simulink model "question1"  (R2019a)
settings: Solver=VariableStepAuto  StartTime=0.0  StopTime=3  RelTol=1e-3
libraries: fl_lib x69, nesl_utility x22
settings Model: Creator=11lot  LastModifiedBy=11lot

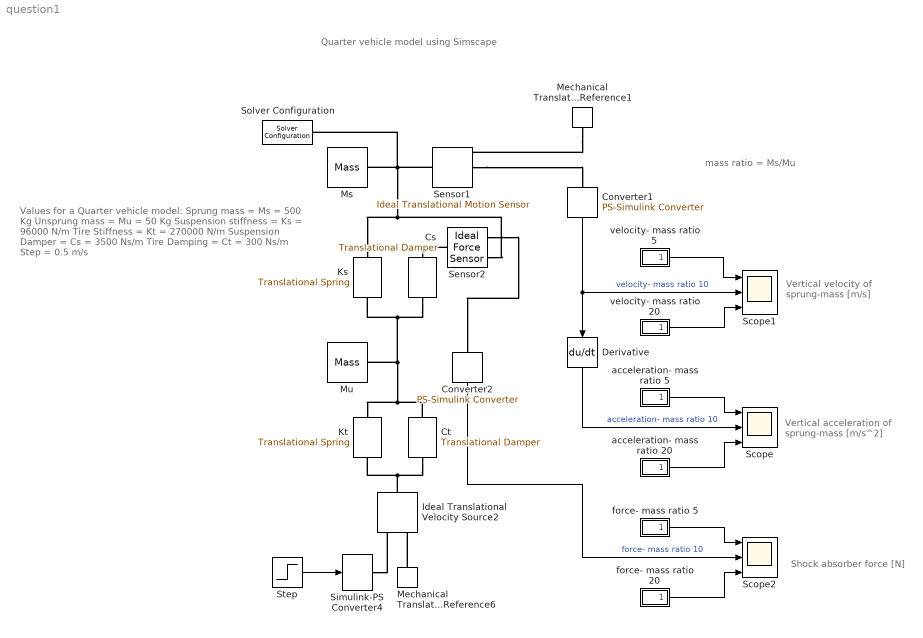
== system question1 ==
  note: mass ratio = Ms/Mu
  note: Values for a Quarter vehicle model:
      |
      | Sprung mass = Ms = 500 Kg
      | Unsprung mass = Mu = 50 Kg
      | Suspension stiffness = Ks = 96000 N/m
      | Tire Stiffness = Kt = 270000 N/m
      | Suspension Damper = Cs = 3500 Ns/m
      | Tire Damping = Ct = 300 Ns/m
      | Step = 0.5 m/s
  note: Quarter vehicle model using Simscape
  note: Vertical velocity of sprung-mass [m/s]
  note: Vertical acceleration of sprung-mass [m/s^2]
  note: Shock absorber force [N]
  " Ks" : fl_lib/Mechanical/Translational Elements/Translational Spring  spr_rate=96000 N/m  v_specify=off  v_priority=High  v=0 m/s  v_nominal_specify=off  v_nominal_unit=m/s  v_nominal_value=1  f_specify=off  f_priority=None  f=0 N  f_nominal_specify=off  f_nominal_unit=N  f_nominal_value=1  x_specify=on  x_priority=High  x=0 m  x_nominal_specify=off  x_nominal_unit=m  x_nominal_value=1
  " Kt" : fl_lib/Mechanical/Translational Elements/Translational Spring  spr_rate=270000 N/m  v_specify=off  v_priority=High  v=0 m/s  v_nominal_specify=off  v_nominal_unit=m/s  v_nominal_value=1  f_specify=off  f_priority=None  f=0 N  f_nominal_specify=off  f_nominal_unit=N  f_nominal_value=1  x_specify=on  x_priority=High  x=0 m  x_nominal_specify=off  x_nominal_unit=m  x_nominal_value=1
  " acceleration- mass ratio 20" : Subsystem
  " acceleration- mass ratio 5" : Subsystem
  Converter1 : nesl_utility/PS-Simulink Converter  PhysicalDomain=network_engine_domain  SubClassName=ps_output  LeftPortType=input  RightPortType=output  PseudoPeriodic=off  Frequencies=[]  Unit=m/s  AffineConversion=off
  Converter2 : nesl_utility/PS-Simulink Converter  PhysicalDomain=network_engine_domain  SubClassName=ps_output  LeftPortType=input  RightPortType=output  PseudoPeriodic=off  Frequencies=[]  Unit=N  AffineConversion=off
  Cs : fl_lib/Mechanical/Translational Elements/Translational Damper  D=3500 N/(m/s)  v_specify=off  v_priority=High  v=0 m/s  v_nominal_specify=off  v_nominal_unit=m/s  v_nominal_value=1  f_specify=off  f_priority=None  f=0 N  f_nominal_specify=off  f_nominal_unit=N  f_nominal_value=1
  Ct : fl_lib/Mechanical/Translational Elements/Translational Damper  D=300 N/(m/s)  v_specify=off  v_priority=High  v=0 m/s  v_nominal_specify=off  v_nominal_unit=m/s  v_nominal_value=1  f_specify=off  f_priority=None  f=0 N  f_nominal_specify=off  f_nominal_unit=N  f_nominal_value=1
  Derivative : Derivative
  Ideal Translational Velocity Source2 : fl_lib/Mechanical/Mechanical Sources/Ideal Translational Velocity Source
  Mechanical Translational Reference1 : fl_lib/Mechanical/Translational Elements/Mechanical Translational Reference
  Mechanical Translational Reference6 : fl_lib/Mechanical/Translational Elements/Mechanical Translational Reference
  Ms : fl_lib/Mechanical/Translational Elements/Mass  mass=500 kg  v_specify=on  v_priority=High  v=0 m/s  v_nominal_specify=off  v_nominal_unit=m/s  v_nominal_value=1  f_specify=off  f_priority=High  f=0 N  f_nominal_specify=off  f_nominal_unit=N  f_nominal_value=1
  Mu : fl_lib/Mechanical/Translational Elements/Mass  mass=50 kg  v_specify=on  v_priority=High  v=0 m/s  v_nominal_specify=off  v_nominal_unit=m/s  v_nominal_value=1  f_specify=off  f_priority=High  f=0 N  f_nominal_specify=off  f_nominal_unit=N  f_nominal_value=1
  Scope : Scope  NumInputPorts=3
  Scope1 : Scope  NumInputPorts=3
  Scope2 : Scope  NumInputPorts=3
  Sensor1 : fl_lib/Mechanical/Mechanical Sensors/Ideal Translational Motion Sensor  offset=0 m
  Sensor2 : fl_lib/Mechanical/Mechanical Sensors/Ideal Force Sensor
  Simulink-PS Converter4 : nesl_utility/Simulink-PS Converter  PhysicalDomain=network_engine_domain  SubClassName=ps_input  LeftPortType=input  RightPortType=output  PseudoPeriodic=off  Frequencies=[]  NoiseDistribution=none  NoiseParameters=[]  Unit=m/s  AffineConversion=off  FilteringAndDerivatives=zero  SimscapeFilterOrder=1  InputFilterTimeConstant=.001  UdotUserProvided=1
  Solver Configuration : nesl_utility/Solver Configuration  PhysicalDomain=network_engine_domain  SubClassName=solver  LeftPortType=input  RightPortType=generic  Tones=[]  Harmonics=[]  SimulateNoise=off  Profile=off  UseLocalSampling=off  EnableSwitchedLinearOptims=on  FrequencyDomain=off  UseCCode=off  RelTol=0.001  AbsTol=1e-06  MinStep=1e-09  ToWorkspace=off  RevertToSquareIcSolve=off  NumHomotopyIterations=100  PhasorMode=off  PhasorModeNumHarmonics=1  DoDC=off  ResidualTolerance=1e-9  UseLocalSolver=off  LocalSolverChoice=NE_BACKWARD_EULER_ADVANCER  LocalSolverSampleTime=.001  DoFixedCost=off  MaxNonlinIter=12  MaxModeIter=2  LinearAlgebra=Sparse  EquationFormulation=NE_TIME_EF  DelaysMemoryBudget=1024  AutomaticFiltering=on  FilteringTimeConstant=0.001  PartitionStorageMethod=AS_NEEDED  PartitionMemoryBudget=1024  PartitionMethod=FAST
  Step : Step  Time=0  After=0.5  SampleTime=0
  force- mass ratio 20 : Subsystem
  force- mass ratio 5 : Subsystem
  velocity- mass ratio 20 : Subsystem
  velocity- mass ratio 5 : Subsystem
  wires:
  Step/1 -> Simulink-PS Converter4/1
  Converter1/1 -> Derivative/1, Scope1/2  "velocity- mass ratio 10"
  Derivative/1 -> Scope/2  "acceleration- mass ratio 10"
  velocity- mass ratio 5/1(Out1) -> Scope1/1
  velocity- mass ratio 20/1(Out2) -> Scope1/3
  " acceleration- mass ratio 5"/1(Out1) -> Scope/1
  " acceleration- mass ratio 20"/1(Out1) -> Scope/3
  Converter2/1 -> Scope2/2  "force- mass ratio 10"
  force- mass ratio 5/1(Out1) -> Scope2/1
  force- mass ratio 20/1(Out1) -> Scope2/3
  connections:
  " Ks"/RConn1 -- Ct/LConn1 -- " Kt"/LConn1 -- Mu/LConn1 -- Cs/RConn1
  Ideal Translational Velocity Source2/LConn1 -- Ct/RConn1 -- " Kt"/RConn1
  Sensor1/LConn1 -- Solver Configuration/RConn1 -- Ms/LConn1 -- Sensor2/RConn1 -- " Ks"/LConn1
  Mechanical Translational Reference6/LConn1 -- Ideal Translational Velocity Source2/RConn2
  Simulink-PS Converter4/RConn1 -- Ideal Translational Velocity Source2/RConn1
  Mechanical Translational Reference1/LConn1 -- Sensor1/RConn1
  Sensor1/RConn2 -- Converter1/LConn1
  Sensor2/RConn2 -- Converter2/LConn1
  Sensor2/LConn1 -- Cs/LConn1

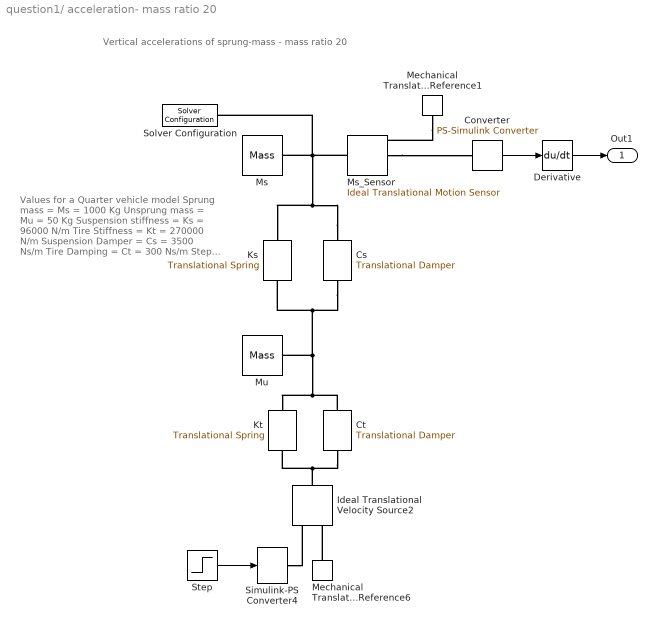
== system question1/ acceleration- mass ratio 20 ==
  note: Vertical accelerations of sprung-mass - mass ratio 20
  note: Values for a Quarter vehicle model
      |
      | Sprung mass = Ms = 1000 Kg
      | Unsprung mass = Mu = 50 Kg
      | Suspension stiffness = Ks = 96000 N/m
      | Tire Stiffness = Kt = 270000 N/m
      | Suspension Damper = Cs = 3500 Ns/m
      | Tire Damping = Ct = 300 Ns/m
      | Step = 0.5 m/s
  " Ms_Sensor" : fl_lib/Mechanical/Mechanical Sensors/Ideal Translational Motion Sensor  offset=0 m
  " Ks" : fl_lib/Mechanical/Translational Elements/Translational Spring  spr_rate=96000 N/m  v_specify=off  v_priority=None  v=0 m/s  v_nominal_specify=off  v_nominal_unit=m/s  v_nominal_value=1  f_specify=off  f_priority=None  f=0 N  f_nominal_specify=off  f_nominal_unit=N  f_nominal_value=1  x_specify=on  x_priority=High  x=0 m  x_nominal_specify=off  x_nominal_unit=m  x_nominal_value=1
  " Kt" : fl_lib/Mechanical/Translational Elements/Translational Spring  spr_rate=270000 N/m  v_specify=off  v_priority=None  v=0 m/s  v_nominal_specify=off  v_nominal_unit=m/s  v_nominal_value=1  f_specify=off  f_priority=None  f=0 N  f_nominal_specify=off  f_nominal_unit=N  f_nominal_value=1  x_specify=on  x_priority=High  x=0 m  x_nominal_specify=off  x_nominal_unit=m  x_nominal_value=1
  Converter : nesl_utility/PS-Simulink Converter  PhysicalDomain=network_engine_domain  SubClassName=ps_output  LeftPortType=input  RightPortType=output  PseudoPeriodic=off  Frequencies=[]  Unit=m/s  AffineConversion=off
  Cs : fl_lib/Mechanical/Translational Elements/Translational Damper  D=3500 N/(m/s)  v_specify=off  v_priority=None  v=0 m/s  v_nominal_specify=off  v_nominal_unit=m/s  v_nominal_value=1  f_specify=off  f_priority=None  f=0 N  f_nominal_specify=off  f_nominal_unit=N  f_nominal_value=1
  Ct : fl_lib/Mechanical/Translational Elements/Translational Damper  D=300 N/(m/s)  v_specify=off  v_priority=None  v=0 m/s  v_nominal_specify=off  v_nominal_unit=m/s  v_nominal_value=1  f_specify=off  f_priority=None  f=0 N  f_nominal_specify=off  f_nominal_unit=N  f_nominal_value=1
  Derivative : Derivative
  Ideal Translational Velocity Source2 : fl_lib/Mechanical/Mechanical Sources/Ideal Translational Velocity Source
  Mechanical Translational Reference1 : fl_lib/Mechanical/Translational Elements/Mechanical Translational Reference
  Mechanical Translational Reference6 : fl_lib/Mechanical/Translational Elements/Mechanical Translational Reference
  Ms : fl_lib/Mechanical/Translational Elements/Mass  mass=1000 kg  v_specify=on  v_priority=High  v=0 m/s  v_nominal_specify=off  v_nominal_unit=m/s  v_nominal_value=1  f_specify=off  f_priority=None  f=0 N  f_nominal_specify=off  f_nominal_unit=N  f_nominal_value=1
  Mu : fl_lib/Mechanical/Translational Elements/Mass  mass=50 kg  v_specify=on  v_priority=High  v=0 m/s  v_nominal_specify=off  v_nominal_unit=m/s  v_nominal_value=1  f_specify=off  f_priority=None  f=0 N  f_nominal_specify=off  f_nominal_unit=N  f_nominal_value=1
  Simulink-PS Converter4 : nesl_utility/Simulink-PS Converter  PhysicalDomain=network_engine_domain  SubClassName=ps_input  LeftPortType=input  RightPortType=output  PseudoPeriodic=off  Frequencies=[]  NoiseDistribution=none  NoiseParameters=[]  Unit=m/s  AffineConversion=off  FilteringAndDerivatives=zero  SimscapeFilterOrder=1  InputFilterTimeConstant=.001  UdotUserProvided=1
  Solver Configuration : nesl_utility/Solver Configuration  PhysicalDomain=network_engine_domain  SubClassName=solver  LeftPortType=input  RightPortType=generic  Tones=[]  Harmonics=[]  SimulateNoise=off  Profile=off  UseLocalSampling=off  EnableSwitchedLinearOptims=on  FrequencyDomain=off  UseCCode=off  RelTol=0.001  AbsTol=1e-06  MinStep=1e-09  ToWorkspace=off  RevertToSquareIcSolve=off  NumHomotopyIterations=100  PhasorMode=off  PhasorModeNumHarmonics=1  DoDC=off  ResidualTolerance=1e-9  UseLocalSolver=off  LocalSolverChoice=NE_BACKWARD_EULER_ADVANCER  LocalSolverSampleTime=.001  DoFixedCost=off  MaxNonlinIter=12  MaxModeIter=2  LinearAlgebra=Sparse  EquationFormulation=NE_TIME_EF  DelaysMemoryBudget=1024  AutomaticFiltering=on  FilteringTimeConstant=0.001  PartitionStorageMethod=AS_NEEDED  PartitionMemoryBudget=1024  PartitionMethod=FAST
  Step : Step  Time=0  After=0.5  SampleTime=0
  Out1 : Outport
  wires:
  Step/1 -> Simulink-PS Converter4/1
  Converter/1 -> Derivative/1
  Derivative/1 -> Out1/1
  connections:
  Ct/LConn1 -- " Kt"/LConn1 -- Mu/LConn1 -- Cs/RConn1 -- " Ks"/RConn1
  Cs/LConn1 -- " Ms_Sensor"/LConn1 -- Solver Configuration/RConn1 -- Ms/LConn1 -- " Ks"/LConn1
  " Kt"/RConn1 -- Ct/RConn1 -- Ideal Translational Velocity Source2/LConn1
  " Ms_Sensor"/RConn2 -- Converter/LConn1
  Mechanical Translational Reference1/LConn1 -- " Ms_Sensor"/RConn1
  Mechanical Translational Reference6/LConn1 -- Ideal Translational Velocity Source2/RConn2
  Simulink-PS Converter4/RConn1 -- Ideal Translational Velocity Source2/RConn1

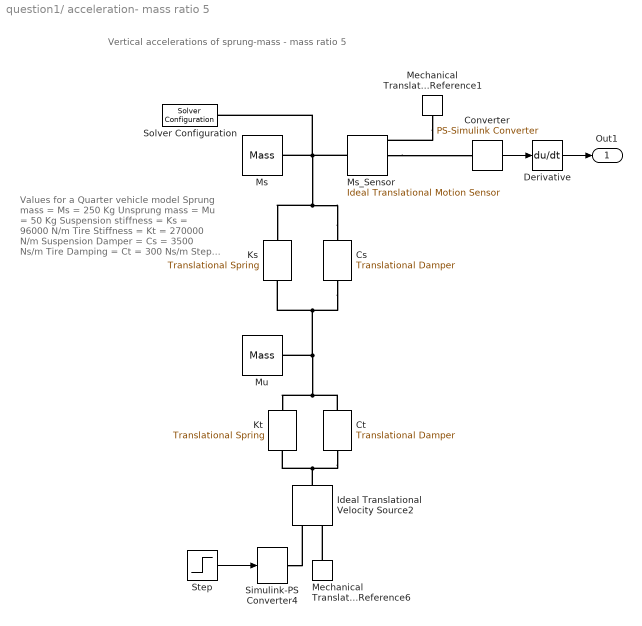
== system question1/ acceleration- mass ratio 5 ==
  note: Vertical accelerations of sprung-mass - mass ratio 5
  note: Values for a Quarter vehicle model
      |
      | Sprung mass = Ms = 250 Kg
      | Unsprung mass = Mu = 50 Kg
      | Suspension stiffness = Ks = 96000 N/m
      | Tire Stiffness = Kt = 270000 N/m
      | Suspension Damper = Cs = 3500 Ns/m
      | Tire Damping = Ct = 300 Ns/m
      | Step = 0.5 m/s
  " Ms_Sensor" : fl_lib/Mechanical/Mechanical Sensors/Ideal Translational Motion Sensor  offset=0 m
  " Ks" : fl_lib/Mechanical/Translational Elements/Translational Spring  spr_rate=96000 N/m  v_specify=off  v_priority=None  v=0 m/s  v_nominal_specify=off  v_nominal_unit=m/s  v_nominal_value=1  f_specify=off  f_priority=None  f=0 N  f_nominal_specify=off  f_nominal_unit=N  f_nominal_value=1  x_specify=on  x_priority=High  x=0 m  x_nominal_specify=off  x_nominal_unit=m  x_nominal_value=1
  " Kt" : fl_lib/Mechanical/Translational Elements/Translational Spring  spr_rate=270000 N/m  v_specify=off  v_priority=None  v=0 m/s  v_nominal_specify=off  v_nominal_unit=m/s  v_nominal_value=1  f_specify=off  f_priority=None  f=0 N  f_nominal_specify=off  f_nominal_unit=N  f_nominal_value=1  x_specify=on  x_priority=High  x=0 m  x_nominal_specify=off  x_nominal_unit=m  x_nominal_value=1
  Converter : nesl_utility/PS-Simulink Converter  PhysicalDomain=network_engine_domain  SubClassName=ps_output  LeftPortType=input  RightPortType=output  PseudoPeriodic=off  Frequencies=[]  Unit=m/s  AffineConversion=off
  Cs : fl_lib/Mechanical/Translational Elements/Translational Damper  D=3500 N/(m/s)  v_specify=off  v_priority=None  v=0 m/s  v_nominal_specify=off  v_nominal_unit=m/s  v_nominal_value=1  f_specify=off  f_priority=None  f=0 N  f_nominal_specify=off  f_nominal_unit=N  f_nominal_value=1
  Ct : fl_lib/Mechanical/Translational Elements/Translational Damper  D=300 N/(m/s)  v_specify=off  v_priority=None  v=0 m/s  v_nominal_specify=off  v_nominal_unit=m/s  v_nominal_value=1  f_specify=off  f_priority=None  f=0 N  f_nominal_specify=off  f_nominal_unit=N  f_nominal_value=1
  Derivative : Derivative
  Ideal Translational Velocity Source2 : fl_lib/Mechanical/Mechanical Sources/Ideal Translational Velocity Source
  Mechanical Translational Reference1 : fl_lib/Mechanical/Translational Elements/Mechanical Translational Reference
  Mechanical Translational Reference6 : fl_lib/Mechanical/Translational Elements/Mechanical Translational Reference
  Ms : fl_lib/Mechanical/Translational Elements/Mass  mass=250 kg  v_specify=on  v_priority=High  v=0 m/s  v_nominal_specify=off  v_nominal_unit=m/s  v_nominal_value=1  f_specify=off  f_priority=None  f=0 N  f_nominal_specify=off  f_nominal_unit=N  f_nominal_value=1
  Mu : fl_lib/Mechanical/Translational Elements/Mass  mass=50 kg  v_specify=on  v_priority=High  v=0 m/s  v_nominal_specify=off  v_nominal_unit=m/s  v_nominal_value=1  f_specify=off  f_priority=None  f=0 N  f_nominal_specify=off  f_nominal_unit=N  f_nominal_value=1
  Simulink-PS Converter4 : nesl_utility/Simulink-PS Converter  PhysicalDomain=network_engine_domain  SubClassName=ps_input  LeftPortType=input  RightPortType=output  PseudoPeriodic=off  Frequencies=[]  NoiseDistribution=none  NoiseParameters=[]  Unit=m/s  AffineConversion=off  FilteringAndDerivatives=zero  SimscapeFilterOrder=1  InputFilterTimeConstant=.001  UdotUserProvided=1
  Solver Configuration : nesl_utility/Solver Configuration  PhysicalDomain=network_engine_domain  SubClassName=solver  LeftPortType=input  RightPortType=generic  Tones=[]  Harmonics=[]  SimulateNoise=off  Profile=off  UseLocalSampling=off  EnableSwitchedLinearOptims=on  FrequencyDomain=off  UseCCode=off  RelTol=0.001  AbsTol=1e-06  MinStep=1e-09  ToWorkspace=off  RevertToSquareIcSolve=off  NumHomotopyIterations=100  PhasorMode=off  PhasorModeNumHarmonics=1  DoDC=off  ResidualTolerance=1e-9  UseLocalSolver=off  LocalSolverChoice=NE_BACKWARD_EULER_ADVANCER  LocalSolverSampleTime=.001  DoFixedCost=off  MaxNonlinIter=12  MaxModeIter=2  LinearAlgebra=Sparse  EquationFormulation=NE_TIME_EF  DelaysMemoryBudget=1024  AutomaticFiltering=on  FilteringTimeConstant=0.001  PartitionStorageMethod=AS_NEEDED  PartitionMemoryBudget=1024  PartitionMethod=FAST
  Step : Step  Time=0  After=0.5  SampleTime=0
  Out1 : Outport
  wires:
  Step/1 -> Simulink-PS Converter4/1
  Converter/1 -> Derivative/1
  Derivative/1 -> Out1/1
  connections:
  Ct/LConn1 -- " Kt"/LConn1 -- Mu/LConn1 -- Cs/RConn1 -- " Ks"/RConn1
  Cs/LConn1 -- " Ms_Sensor"/LConn1 -- Solver Configuration/RConn1 -- Ms/LConn1 -- " Ks"/LConn1
  " Kt"/RConn1 -- Ct/RConn1 -- Ideal Translational Velocity Source2/LConn1
  " Ms_Sensor"/RConn2 -- Converter/LConn1
  Mechanical Translational Reference1/LConn1 -- " Ms_Sensor"/RConn1
  Mechanical Translational Reference6/LConn1 -- Ideal Translational Velocity Source2/RConn2
  Simulink-PS Converter4/RConn1 -- Ideal Translational Velocity Source2/RConn1

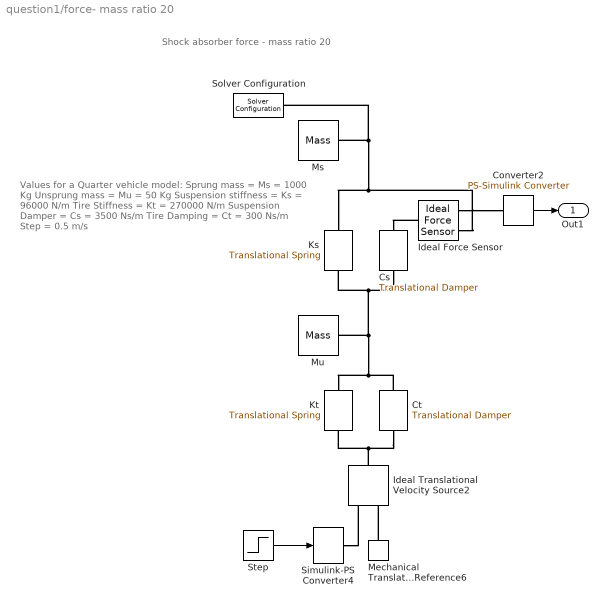
== system question1/force- mass ratio 20 ==
  note: Shock absorber force - mass ratio 20
  note: Values for a Quarter vehicle model:
      |
      | Sprung mass = Ms = 1000 Kg
      | Unsprung mass = Mu = 50 Kg
      | Suspension stiffness = Ks = 96000 N/m
      | Tire Stiffness = Kt = 270000 N/m
      | Suspension Damper = Cs = 3500 Ns/m
      | Tire Damping = Ct = 300 Ns/m
      | Step = 0.5 m/s
  " Ks" : fl_lib/Mechanical/Translational Elements/Translational Spring  spr_rate=96000 N/m  v_specify=off  v_priority=High  v=0 m/s  v_nominal_specify=off  v_nominal_unit=m/s  v_nominal_value=1  f_specify=off  f_priority=None  f=0 N  f_nominal_specify=off  f_nominal_unit=N  f_nominal_value=1  x_specify=on  x_priority=High  x=0 m  x_nominal_specify=off  x_nominal_unit=m  x_nominal_value=1
  " Kt" : fl_lib/Mechanical/Translational Elements/Translational Spring  spr_rate=270000 N/m  v_specify=off  v_priority=High  v=0 m/s  v_nominal_specify=off  v_nominal_unit=m/s  v_nominal_value=1  f_specify=off  f_priority=None  f=0 N  f_nominal_specify=off  f_nominal_unit=N  f_nominal_value=1  x_specify=on  x_priority=High  x=0 m  x_nominal_specify=off  x_nominal_unit=m  x_nominal_value=1
  Converter2 : nesl_utility/PS-Simulink Converter  PhysicalDomain=network_engine_domain  SubClassName=ps_output  LeftPortType=input  RightPortType=output  PseudoPeriodic=off  Frequencies=[]  Unit=N  AffineConversion=off
  Cs : fl_lib/Mechanical/Translational Elements/Translational Damper  D=3500 N/(m/s)  v_specify=off  v_priority=High  v=0 m/s  v_nominal_specify=off  v_nominal_unit=m/s  v_nominal_value=1  f_specify=off  f_priority=None  f=0 N  f_nominal_specify=off  f_nominal_unit=N  f_nominal_value=1
  Ct : fl_lib/Mechanical/Translational Elements/Translational Damper  D=300 N/(m/s)  v_specify=off  v_priority=High  v=0 m/s  v_nominal_specify=off  v_nominal_unit=m/s  v_nominal_value=1  f_specify=off  f_priority=None  f=0 N  f_nominal_specify=off  f_nominal_unit=N  f_nominal_value=1
  Ideal Force Sensor : fl_lib/Mechanical/Mechanical Sensors/Ideal Force Sensor
  Ideal Translational Velocity Source2 : fl_lib/Mechanical/Mechanical Sources/Ideal Translational Velocity Source
  Mechanical Translational Reference6 : fl_lib/Mechanical/Translational Elements/Mechanical Translational Reference
  Ms : fl_lib/Mechanical/Translational Elements/Mass  mass=1000 kg  v_specify=on  v_priority=High  v=0 m/s  v_nominal_specify=off  v_nominal_unit=m/s  v_nominal_value=1  f_specify=off  f_priority=High  f=0 N  f_nominal_specify=off  f_nominal_unit=N  f_nominal_value=1
  Mu : fl_lib/Mechanical/Translational Elements/Mass  mass=50 kg  v_specify=on  v_priority=High  v=0 m/s  v_nominal_specify=off  v_nominal_unit=m/s  v_nominal_value=1  f_specify=off  f_priority=High  f=0 N  f_nominal_specify=off  f_nominal_unit=N  f_nominal_value=1
  Simulink-PS Converter4 : nesl_utility/Simulink-PS Converter  PhysicalDomain=network_engine_domain  SubClassName=ps_input  LeftPortType=input  RightPortType=output  PseudoPeriodic=off  Frequencies=[]  NoiseDistribution=none  NoiseParameters=[]  Unit=m/s  AffineConversion=off  FilteringAndDerivatives=zero  SimscapeFilterOrder=1  InputFilterTimeConstant=.001  UdotUserProvided=1
  Solver Configuration : nesl_utility/Solver Configuration  PhysicalDomain=network_engine_domain  SubClassName=solver  LeftPortType=input  RightPortType=generic  Tones=[]  Harmonics=[]  SimulateNoise=off  Profile=off  UseLocalSampling=off  EnableSwitchedLinearOptims=on  FrequencyDomain=off  UseCCode=off  RelTol=0.001  AbsTol=1e-06  MinStep=1e-09  ToWorkspace=off  RevertToSquareIcSolve=off  NumHomotopyIterations=100  PhasorMode=off  PhasorModeNumHarmonics=1  DoDC=off  ResidualTolerance=1e-9  UseLocalSolver=off  LocalSolverChoice=NE_BACKWARD_EULER_ADVANCER  LocalSolverSampleTime=.001  DoFixedCost=off  MaxNonlinIter=12  MaxModeIter=2  LinearAlgebra=Sparse  EquationFormulation=NE_TIME_EF  DelaysMemoryBudget=1024  AutomaticFiltering=on  FilteringTimeConstant=0.001  PartitionStorageMethod=AS_NEEDED  PartitionMemoryBudget=1024  PartitionMethod=FAST
  Step : Step  Time=0  After=0.5  SampleTime=0
  Out1 : Outport
  wires:
  Converter2/1 -> Out1/1
  Step/1 -> Simulink-PS Converter4/1
  connections:
  Cs/RConn1 -- " Ks"/RConn1 -- Ct/LConn1 -- " Kt"/LConn1 -- Mu/LConn1
  Ideal Force Sensor/RConn1 -- " Ks"/LConn1 -- Solver Configuration/RConn1 -- Ms/LConn1
  Ct/RConn1 -- " Kt"/RConn1 -- Ideal Translational Velocity Source2/LConn1
  Ideal Force Sensor/LConn1 -- Cs/LConn1
  Simulink-PS Converter4/RConn1 -- Ideal Translational Velocity Source2/RConn1
  Mechanical Translational Reference6/LConn1 -- Ideal Translational Velocity Source2/RConn2
  Ideal Force Sensor/RConn2 -- Converter2/LConn1

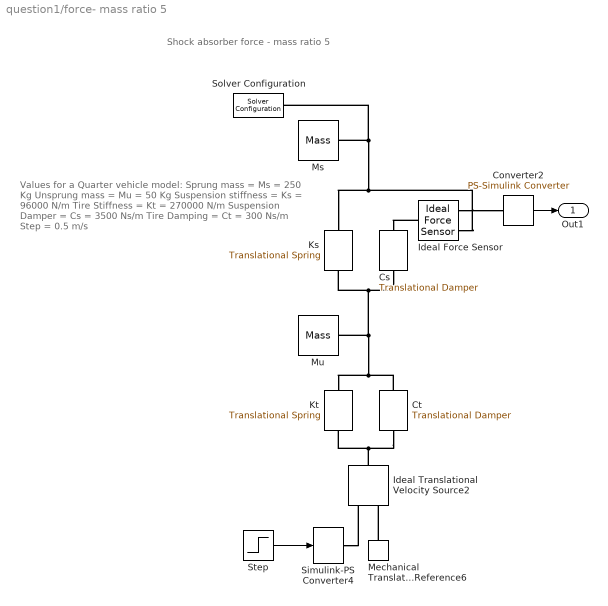
== system question1/force- mass ratio 5 ==
  note: Shock absorber force - mass ratio 5
  note: Values for a Quarter vehicle model:
      |
      | Sprung mass = Ms = 250 Kg
      | Unsprung mass = Mu = 50 Kg
      | Suspension stiffness = Ks = 96000 N/m
      | Tire Stiffness = Kt = 270000 N/m
      | Suspension Damper = Cs = 3500 Ns/m
      | Tire Damping = Ct = 300 Ns/m
      | Step = 0.5 m/s
  " Ks" : fl_lib/Mechanical/Translational Elements/Translational Spring  spr_rate=96000 N/m  v_specify=off  v_priority=High  v=0 m/s  v_nominal_specify=off  v_nominal_unit=m/s  v_nominal_value=1  f_specify=off  f_priority=None  f=0 N  f_nominal_specify=off  f_nominal_unit=N  f_nominal_value=1  x_specify=on  x_priority=High  x=0 m  x_nominal_specify=off  x_nominal_unit=m  x_nominal_value=1
  " Kt" : fl_lib/Mechanical/Translational Elements/Translational Spring  spr_rate=270000 N/m  v_specify=off  v_priority=High  v=0 m/s  v_nominal_specify=off  v_nominal_unit=m/s  v_nominal_value=1  f_specify=off  f_priority=None  f=0 N  f_nominal_specify=off  f_nominal_unit=N  f_nominal_value=1  x_specify=on  x_priority=High  x=0 m  x_nominal_specify=off  x_nominal_unit=m  x_nominal_value=1
  Converter2 : nesl_utility/PS-Simulink Converter  PhysicalDomain=network_engine_domain  SubClassName=ps_output  LeftPortType=input  RightPortType=output  PseudoPeriodic=off  Frequencies=[]  Unit=N  AffineConversion=off
  Cs : fl_lib/Mechanical/Translational Elements/Translational Damper  D=3500 N/(m/s)  v_specify=off  v_priority=High  v=0 m/s  v_nominal_specify=off  v_nominal_unit=m/s  v_nominal_value=1  f_specify=off  f_priority=None  f=0 N  f_nominal_specify=off  f_nominal_unit=N  f_nominal_value=1
  Ct : fl_lib/Mechanical/Translational Elements/Translational Damper  D=300 N/(m/s)  v_specify=off  v_priority=High  v=0 m/s  v_nominal_specify=off  v_nominal_unit=m/s  v_nominal_value=1  f_specify=off  f_priority=None  f=0 N  f_nominal_specify=off  f_nominal_unit=N  f_nominal_value=1
  Ideal Force Sensor : fl_lib/Mechanical/Mechanical Sensors/Ideal Force Sensor
  Ideal Translational Velocity Source2 : fl_lib/Mechanical/Mechanical Sources/Ideal Translational Velocity Source
  Mechanical Translational Reference6 : fl_lib/Mechanical/Translational Elements/Mechanical Translational Reference
  Ms : fl_lib/Mechanical/Translational Elements/Mass  mass=250 kg  v_specify=on  v_priority=High  v=0 m/s  v_nominal_specify=off  v_nominal_unit=m/s  v_nominal_value=1  f_specify=off  f_priority=High  f=0 N  f_nominal_specify=off  f_nominal_unit=N  f_nominal_value=1
  Mu : fl_lib/Mechanical/Translational Elements/Mass  mass=50 kg  v_specify=on  v_priority=High  v=0 m/s  v_nominal_specify=off  v_nominal_unit=m/s  v_nominal_value=1  f_specify=off  f_priority=High  f=0 N  f_nominal_specify=off  f_nominal_unit=N  f_nominal_value=1
  Simulink-PS Converter4 : nesl_utility/Simulink-PS Converter  PhysicalDomain=network_engine_domain  SubClassName=ps_input  LeftPortType=input  RightPortType=output  PseudoPeriodic=off  Frequencies=[]  NoiseDistribution=none  NoiseParameters=[]  Unit=m/s  AffineConversion=off  FilteringAndDerivatives=zero  SimscapeFilterOrder=1  InputFilterTimeConstant=.001  UdotUserProvided=1
  Solver Configuration : nesl_utility/Solver Configuration  PhysicalDomain=network_engine_domain  SubClassName=solver  LeftPortType=input  RightPortType=generic  Tones=[]  Harmonics=[]  SimulateNoise=off  Profile=off  UseLocalSampling=off  EnableSwitchedLinearOptims=on  FrequencyDomain=off  UseCCode=off  RelTol=0.001  AbsTol=1e-06  MinStep=1e-09  ToWorkspace=off  RevertToSquareIcSolve=off  NumHomotopyIterations=100  PhasorMode=off  PhasorModeNumHarmonics=1  DoDC=off  ResidualTolerance=1e-9  UseLocalSolver=off  LocalSolverChoice=NE_BACKWARD_EULER_ADVANCER  LocalSolverSampleTime=.001  DoFixedCost=off  MaxNonlinIter=12  MaxModeIter=2  LinearAlgebra=Sparse  EquationFormulation=NE_TIME_EF  DelaysMemoryBudget=1024  AutomaticFiltering=on  FilteringTimeConstant=0.001  PartitionStorageMethod=AS_NEEDED  PartitionMemoryBudget=1024  PartitionMethod=FAST
  Step : Step  Time=0  After=0.5  SampleTime=0
  Out1 : Outport
  wires:
  Converter2/1 -> Out1/1
  Step/1 -> Simulink-PS Converter4/1
  connections:
  " Ks"/RConn1 -- Ct/LConn1 -- " Kt"/LConn1 -- Mu/LConn1 -- Cs/RConn1
  Ms/LConn1 -- Ideal Force Sensor/RConn1 -- " Ks"/LConn1 -- Solver Configuration/RConn1
  " Kt"/RConn1 -- Ideal Translational Velocity Source2/LConn1 -- Ct/RConn1
  Ideal Force Sensor/LConn1 -- Cs/LConn1
  Simulink-PS Converter4/RConn1 -- Ideal Translational Velocity Source2/RConn1
  Mechanical Translational Reference6/LConn1 -- Ideal Translational Velocity Source2/RConn2
  Ideal Force Sensor/RConn2 -- Converter2/LConn1

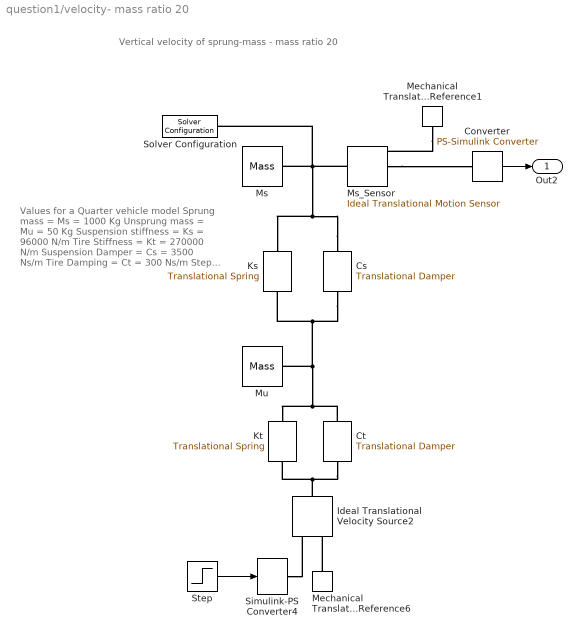
== system question1/velocity- mass ratio 20 ==
  note: Vertical velocity of sprung-mass - mass ratio 20
  note: Values for a Quarter vehicle model
      |
      | Sprung mass = Ms = 1000 Kg
      | Unsprung mass = Mu = 50 Kg
      | Suspension stiffness = Ks = 96000 N/m
      | Tire Stiffness = Kt = 270000 N/m
      | Suspension Damper = Cs = 3500 Ns/m
      | Tire Damping = Ct = 300 Ns/m
      | Step = 0.5 m/s
  " Ms_Sensor" : fl_lib/Mechanical/Mechanical Sensors/Ideal Translational Motion Sensor  offset=0 m
  " Ks" : fl_lib/Mechanical/Translational Elements/Translational Spring  spr_rate=96000 N/m  v_specify=off  v_priority=None  v=0 m/s  v_nominal_specify=off  v_nominal_unit=m/s  v_nominal_value=1  f_specify=off  f_priority=None  f=0 N  f_nominal_specify=off  f_nominal_unit=N  f_nominal_value=1  x_specify=on  x_priority=High  x=0 m  x_nominal_specify=off  x_nominal_unit=m  x_nominal_value=1
  " Kt" : fl_lib/Mechanical/Translational Elements/Translational Spring  spr_rate=270000 N/m  v_specify=off  v_priority=None  v=0 m/s  v_nominal_specify=off  v_nominal_unit=m/s  v_nominal_value=1  f_specify=off  f_priority=None  f=0 N  f_nominal_specify=off  f_nominal_unit=N  f_nominal_value=1  x_specify=on  x_priority=High  x=0 m  x_nominal_specify=off  x_nominal_unit=m  x_nominal_value=1
  Converter : nesl_utility/PS-Simulink Converter  PhysicalDomain=network_engine_domain  SubClassName=ps_output  LeftPortType=input  RightPortType=output  PseudoPeriodic=off  Frequencies=[]  Unit=m/s  AffineConversion=off
  Cs : fl_lib/Mechanical/Translational Elements/Translational Damper  D=3500 N/(m/s)  v_specify=off  v_priority=None  v=0 m/s  v_nominal_specify=off  v_nominal_unit=m/s  v_nominal_value=1  f_specify=off  f_priority=None  f=0 N  f_nominal_specify=off  f_nominal_unit=N  f_nominal_value=1
  Ct : fl_lib/Mechanical/Translational Elements/Translational Damper  D=300 N/(m/s)  v_specify=off  v_priority=None  v=0 m/s  v_nominal_specify=off  v_nominal_unit=m/s  v_nominal_value=1  f_specify=off  f_priority=None  f=0 N  f_nominal_specify=off  f_nominal_unit=N  f_nominal_value=1
  Ideal Translational Velocity Source2 : fl_lib/Mechanical/Mechanical Sources/Ideal Translational Velocity Source
  Mechanical Translational Reference1 : fl_lib/Mechanical/Translational Elements/Mechanical Translational Reference
  Mechanical Translational Reference6 : fl_lib/Mechanical/Translational Elements/Mechanical Translational Reference
  Ms : fl_lib/Mechanical/Translational Elements/Mass  mass=1000 kg  v_specify=on  v_priority=High  v=0 m/s  v_nominal_specify=off  v_nominal_unit=m/s  v_nominal_value=1  f_specify=off  f_priority=None  f=0 N  f_nominal_specify=off  f_nominal_unit=N  f_nominal_value=1
  Mu : fl_lib/Mechanical/Translational Elements/Mass  mass=50 kg  v_specify=on  v_priority=High  v=0 m/s  v_nominal_specify=off  v_nominal_unit=m/s  v_nominal_value=1  f_specify=off  f_priority=None  f=0 N  f_nominal_specify=off  f_nominal_unit=N  f_nominal_value=1
  Simulink-PS Converter4 : nesl_utility/Simulink-PS Converter  PhysicalDomain=network_engine_domain  SubClassName=ps_input  LeftPortType=input  RightPortType=output  PseudoPeriodic=off  Frequencies=[]  NoiseDistribution=none  NoiseParameters=[]  Unit=m/s  AffineConversion=off  FilteringAndDerivatives=zero  SimscapeFilterOrder=1  InputFilterTimeConstant=.001  UdotUserProvided=1
  Solver Configuration : nesl_utility/Solver Configuration  PhysicalDomain=network_engine_domain  SubClassName=solver  LeftPortType=input  RightPortType=generic  Tones=[]  Harmonics=[]  SimulateNoise=off  Profile=off  UseLocalSampling=off  EnableSwitchedLinearOptims=on  FrequencyDomain=off  UseCCode=off  RelTol=0.001  AbsTol=1e-06  MinStep=1e-09  ToWorkspace=off  RevertToSquareIcSolve=off  NumHomotopyIterations=100  PhasorMode=off  PhasorModeNumHarmonics=1  DoDC=off  ResidualTolerance=1e-9  UseLocalSolver=off  LocalSolverChoice=NE_BACKWARD_EULER_ADVANCER  LocalSolverSampleTime=.001  DoFixedCost=off  MaxNonlinIter=12  MaxModeIter=2  LinearAlgebra=Sparse  EquationFormulation=NE_TIME_EF  DelaysMemoryBudget=1024  AutomaticFiltering=on  FilteringTimeConstant=0.001  PartitionStorageMethod=AS_NEEDED  PartitionMemoryBudget=1024  PartitionMethod=FAST
  Step : Step  Time=0  After=0.5  SampleTime=0
  Out2 : Outport
  wires:
  Step/1 -> Simulink-PS Converter4/1
  Converter/1 -> Out2/1
  connections:
  Cs/LConn1 -- " Ks"/LConn1 -- " Ms_Sensor"/LConn1 -- Solver Configuration/RConn1 -- Ms/LConn1
  Ct/RConn1 -- Ideal Translational Velocity Source2/LConn1 -- " Kt"/RConn1
  Cs/RConn1 -- " Ks"/RConn1 -- Mu/LConn1 -- Ct/LConn1 -- " Kt"/LConn1
  Simulink-PS Converter4/RConn1 -- Ideal Translational Velocity Source2/RConn1
  Mechanical Translational Reference1/LConn1 -- " Ms_Sensor"/RConn1
  " Ms_Sensor"/RConn2 -- Converter/LConn1
  Mechanical Translational Reference6/LConn1 -- Ideal Translational Velocity Source2/RConn2

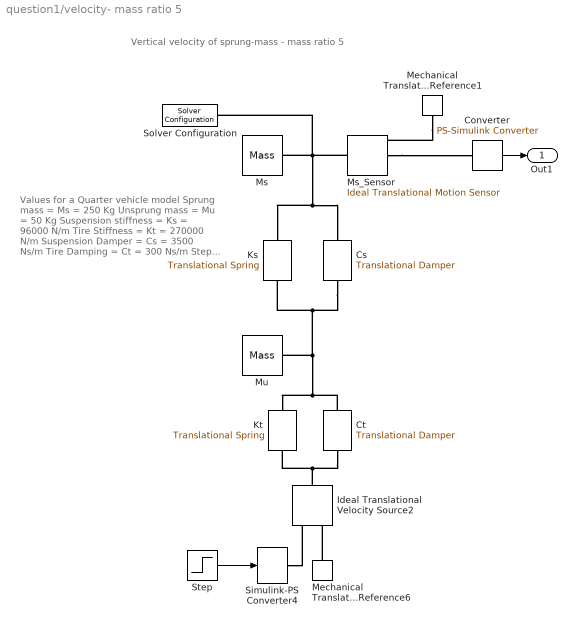
== system question1/velocity- mass ratio 5 ==
  note: Vertical velocity of sprung-mass - mass ratio 5
  note: Values for a Quarter vehicle model
      |
      | Sprung mass = Ms = 250 Kg
      | Unsprung mass = Mu = 50 Kg
      | Suspension stiffness = Ks = 96000 N/m
      | Tire Stiffness = Kt = 270000 N/m
      | Suspension Damper = Cs = 3500 Ns/m
      | Tire Damping = Ct = 300 Ns/m
      | Step = 0.5 m/s
  " Ms_Sensor" : fl_lib/Mechanical/Mechanical Sensors/Ideal Translational Motion Sensor  offset=0 m
  " Ks" : fl_lib/Mechanical/Translational Elements/Translational Spring  spr_rate=96000 N/m  v_specify=off  v_priority=None  v=0 m/s  v_nominal_specify=off  v_nominal_unit=m/s  v_nominal_value=1  f_specify=off  f_priority=None  f=0 N  f_nominal_specify=off  f_nominal_unit=N  f_nominal_value=1  x_specify=on  x_priority=High  x=0 m  x_nominal_specify=off  x_nominal_unit=m  x_nominal_value=1
  " Kt" : fl_lib/Mechanical/Translational Elements/Translational Spring  spr_rate=270000 N/m  v_specify=off  v_priority=None  v=0 m/s  v_nominal_specify=off  v_nominal_unit=m/s  v_nominal_value=1  f_specify=off  f_priority=None  f=0 N  f_nominal_specify=off  f_nominal_unit=N  f_nominal_value=1  x_specify=on  x_priority=High  x=0 m  x_nominal_specify=off  x_nominal_unit=m  x_nominal_value=1
  Converter : nesl_utility/PS-Simulink Converter  PhysicalDomain=network_engine_domain  SubClassName=ps_output  LeftPortType=input  RightPortType=output  PseudoPeriodic=off  Frequencies=[]  Unit=m/s  AffineConversion=off
  Cs : fl_lib/Mechanical/Translational Elements/Translational Damper  D=3500 N/(m/s)  v_specify=off  v_priority=None  v=0 m/s  v_nominal_specify=off  v_nominal_unit=m/s  v_nominal_value=1  f_specify=off  f_priority=None  f=0 N  f_nominal_specify=off  f_nominal_unit=N  f_nominal_value=1
  Ct : fl_lib/Mechanical/Translational Elements/Translational Damper  D=300 N/(m/s)  v_specify=off  v_priority=None  v=0 m/s  v_nominal_specify=off  v_nominal_unit=m/s  v_nominal_value=1  f_specify=off  f_priority=None  f=0 N  f_nominal_specify=off  f_nominal_unit=N  f_nominal_value=1
  Ideal Translational Velocity Source2 : fl_lib/Mechanical/Mechanical Sources/Ideal Translational Velocity Source
  Mechanical Translational Reference1 : fl_lib/Mechanical/Translational Elements/Mechanical Translational Reference
  Mechanical Translational Reference6 : fl_lib/Mechanical/Translational Elements/Mechanical Translational Reference
  Ms : fl_lib/Mechanical/Translational Elements/Mass  mass=250 kg  v_specify=on  v_priority=High  v=0 m/s  v_nominal_specify=off  v_nominal_unit=m/s  v_nominal_value=1  f_specify=off  f_priority=None  f=0 N  f_nominal_specify=off  f_nominal_unit=N  f_nominal_value=1
  Mu : fl_lib/Mechanical/Translational Elements/Mass  mass=50 kg  v_specify=on  v_priority=High  v=0 m/s  v_nominal_specify=off  v_nominal_unit=m/s  v_nominal_value=1  f_specify=off  f_priority=None  f=0 N  f_nominal_specify=off  f_nominal_unit=N  f_nominal_value=1
  Simulink-PS Converter4 : nesl_utility/Simulink-PS Converter  PhysicalDomain=network_engine_domain  SubClassName=ps_input  LeftPortType=input  RightPortType=output  PseudoPeriodic=off  Frequencies=[]  NoiseDistribution=none  NoiseParameters=[]  Unit=m/s  AffineConversion=off  FilteringAndDerivatives=zero  SimscapeFilterOrder=1  InputFilterTimeConstant=.001  UdotUserProvided=1
  Solver Configuration : nesl_utility/Solver Configuration  PhysicalDomain=network_engine_domain  SubClassName=solver  LeftPortType=input  RightPortType=generic  Tones=[]  Harmonics=[]  SimulateNoise=off  Profile=off  UseLocalSampling=off  EnableSwitchedLinearOptims=on  FrequencyDomain=off  UseCCode=off  RelTol=0.001  AbsTol=1e-06  MinStep=1e-09  ToWorkspace=off  RevertToSquareIcSolve=off  NumHomotopyIterations=100  PhasorMode=off  PhasorModeNumHarmonics=1  DoDC=off  ResidualTolerance=1e-9  UseLocalSolver=off  LocalSolverChoice=NE_BACKWARD_EULER_ADVANCER  LocalSolverSampleTime=.001  DoFixedCost=off  MaxNonlinIter=12  MaxModeIter=2  LinearAlgebra=Sparse  EquationFormulation=NE_TIME_EF  DelaysMemoryBudget=1024  AutomaticFiltering=on  FilteringTimeConstant=0.001  PartitionStorageMethod=AS_NEEDED  PartitionMemoryBudget=1024  PartitionMethod=FAST
  Step : Step  Time=0  After=0.5  SampleTime=0
  Out1 : Outport
  wires:
  Converter/1 -> Out1/1
  Step/1 -> Simulink-PS Converter4/1
  connections:
  Cs/RConn1 -- " Ks"/RConn1 -- Ct/LConn1 -- " Kt"/LConn1 -- Mu/LConn1
  Ms/LConn1 -- " Ms_Sensor"/LConn1 -- Solver Configuration/RConn1 -- " Ks"/LConn1 -- Cs/LConn1
  Ct/RConn1 -- Ideal Translational Velocity Source2/LConn1 -- " Kt"/RConn1
  " Ms_Sensor"/RConn2 -- Converter/LConn1
  Mechanical Translational Reference1/LConn1 -- " Ms_Sensor"/RConn1
  Mechanical Translational Reference6/LConn1 -- Ideal Translational Velocity Source2/RConn2
  Simulink-PS Converter4/RConn1 -- Ideal Translational Velocity Source2/RConn1
